simulink model "sampleModel1419"  (R2023a)
settings: Solver=VariableStepAuto  StartTime=0.0  StopTime=10.0  RelTol=1e-3
libraries: hdlsllib x6, simulink x1
settings Model: Creator=user1  LastModifiedBy=user1

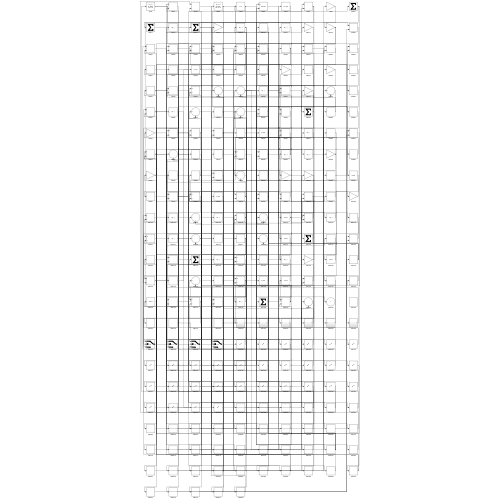
[thumbnail: Simulink's stored preview of the top-level diagram]
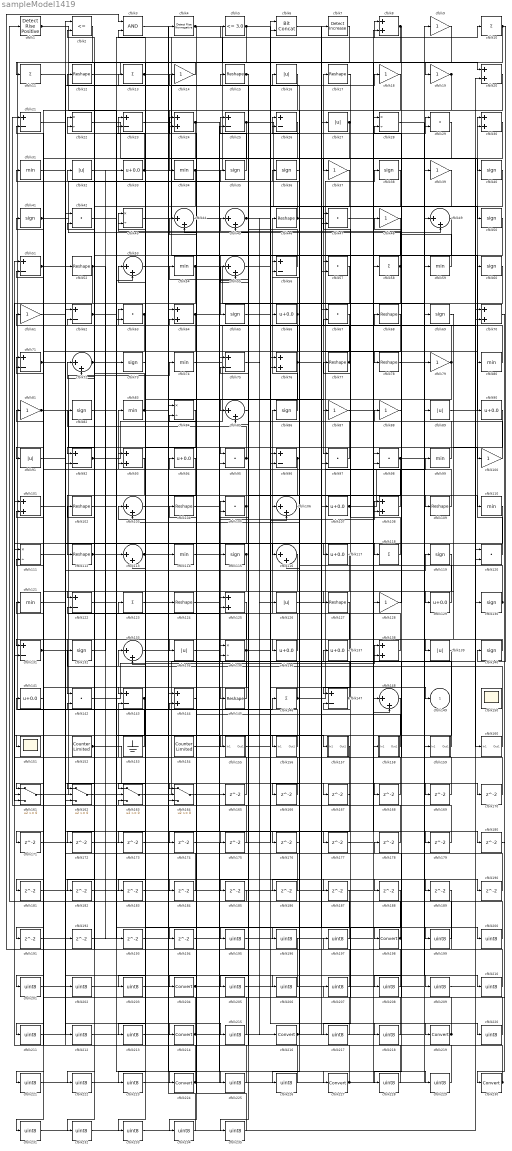
== system sampleModel1419 ==
  cfblk1 : hdlsllib/Logic and Bit Operations/Detect Rise Positive  vinit=0  OutDataTypeStr=boolean
  cfblk{10..11,13,58,118,123,146} (7 alike) : Sum  Inputs=+
  cfblk{9,14,18..19,37,39,48,61,79,81,87..88,100,128} (14 alike) : Gain
  cfblk{8,20,24,30,64,70,76,93,101,108,125,138,144} (13 alike) : Sum
  cfblk{12,15,17,46,52,68,77..78,102,104,109,112,124,127,145} (15 alike) : Reshape
  cfblk{44..45,49,53,55,72,85,103,106,113,116,133,148} (13 alike) : Sum  Inputs=|++
  cfblk{29,42,47,57,63,67,95,97..98,105,120,142} (12 alike) : DotProduct  OutDataTypeStr=Inherit: Inherit via internal rule
  cfblk{33,66,90,94,107,117,129,136..137,141} (10 alike) : Bias  Bias=0.0  SaturateOnIntegerOverflow=off
  cfblk{31,34,54,59,74,80,83,99,110,114,121} (11 alike) : MinMax
  cfblk{22,28,43,84,111,135} (6 alike) : Product  Inputs=*/  RndMeth=Zero  SaturateOnIntegerOverflow=on
  cfblk{35..36,38,40..41,50,60,65,69,73,82,86,115,119,130,132,140} (17 alike) : Signum
  cfblk{21,23,25..26,51,56,62,71,75,92,96,122,131,143,147} (15 alike) : Sum  Inputs=+-
  cfblk{16,27,32,89,91,126,134,139} (8 alike) : Abs  SaturateOnIntegerOverflow=off
  cfblk150 : Scope
      settings: Floating=on
  cfblk151 : Scope
  cfblk152 : hdlsllib/Sources/Counter Limited  uplimit=7  tsamp=-1
  cfblk153 : Ground
  cfblk154 : hdlsllib/Sources/Counter Limited  uplimit=7  tsamp=-1
  cfblk155 : Subsystem
      settings: LibrarySourceBlock=|
      | hdlsllib/Ports &
      | Subsystems/Subsystem
  cfblk156 : Subsystem
      settings: LibrarySourceBlock=|
      | hdlsllib/Ports &
      | Subsystems/Subsystem
  cfblk157 : Subsystem
      settings: LibrarySourceBlock=|
      | hdlsllib/Ports &
      | Subsystems/Subsystem
  cfblk158 : Subsystem
      settings: LibrarySourceBlock=|
      | hdlsllib/Ports &
      | Subsystems/Subsystem
  cfblk159 : Subsystem
      settings: LibrarySourceBlock=|
      | hdlsllib/Ports &
      | Subsystems/Subsystem
  cfblk160 : Subsystem
      settings: LibrarySourceBlock=|
      | hdlsllib/Ports &
      | Subsystems/Subsystem
  cfblk{161..164} (4 alike) : Switch  SaturateOnIntegerOverflow=off  InputSameDT=off
  cfblk{165..194} (30 alike) : Delay  SampleTime=1
  cfblk{195..197,199..203,205..213,215,217..218,220..223,225..226,228..229,231..235} (33 alike) : DataTypeConversion  OutDataTypeStr=uint8  SaturateOnIntegerOverflow=off  RndMeth=Floor
  cfblk{198,204,214,216,219,224,227,230} (8 alike) : DataTypeConversion  SaturateOnIntegerOverflow=off  RndMeth=Floor
  cfblk2 : RelationalOperator  Operator=<=  OutDataTypeStr=boolean  InputSameDT=off
  cfblk3 : Logic  AllPortsSameDT=off  OutDataTypeStr=boolean
  cfblk4 : hdlsllib/Logic and Bit Operations/Detect Rise Nonnegative  vinit=0  OutDataTypeStr=boolean
  cfblk5 : hdlsllib/Logic and Bit Operations/Compare To Constant  relop=<=  const=3.0  OutDataTypeStr=boolean
  cfblk6 : hdlsllib/Logic and Bit Operations/Bit Concat  numInputs=2
  cfblk7 : simulink/Logic and Bit Operations/Detect Increase  vinit=0.0  OutDataTypeStr=boolean
      settings: LibrarySourceBlock=|
      | hdlsllib/Logic and Bit
      | Operations/Detect
      | Increase
  cfblk149 : Outport  VectorParamsAs1DForOutWhenUnconnected=off
  wires:
  cfblk142/1 -> cfblk138/1
  cfblk30/1 -> cfblk156/1(In1)
  cfblk132/1 -> cfblk33/1
  cfblk146/1 -> cfblk38/1, cfblk94/1
  cfblk49/1 -> cfblk65/1
  cfblk43/1 -> cfblk10/1
  cfblk33/1 -> cfblk22/1, cfblk109/1
  cfblk15/1 -> cfblk45/2, cfblk205/1
  cfblk80/1 -> cfblk46/1
  cfblk46/1 -> cfblk18/1, cfblk21/2, cfblk199/1
  cfblk47/1 -> cfblk158/1(In1)
  cfblk50/1 -> cfblk97/1
  cfblk99/1 -> cfblk54/1
  cfblk89/1 -> cfblk30/1
  cfblk2/1 -> cfblk146/1
  cfblk37/1 -> cfblk57/1
  cfblk86/1 -> cfblk66/1
  cfblk113/1 -> cfblk35/1, cfblk167/1
  cfblk42/1 -> cfblk198/1
  cfblk145/1 -> cfblk103/1
  cfblk12/1 -> cfblk20/1
  cfblk120/1 -> cfblk30/2
  cfblk22/1 -> cfblk40/1
  cfblk34/1 -> cfblk8/1, cfblk92/1
  cfblk138/1 -> cfblk86/1
  cfblk147/1 -> cfblk105/1, cfblk122/2
  cfblk107/1 -> cfblk99/1, cfblk147/1
  cfblk105/1 -> cfblk83/1, cfblk131/2
  cfblk13/1 -> cfblk90/1, cfblk37/1
  cfblk109/1 -> cfblk47/1
  cfblk143/1 -> cfblk23/1, cfblk161/3
  cfblk18/1 -> cfblk34/1
  cfblk69/1 -> cfblk139/1
  cfblk158/1(Out1) -> cfblk64/2
  cfblk137/1 -> cfblk63/1
  cfblk126/1 -> cfblk49/1
  cfblk77/1 -> cfblk16/1, cfblk26/1
  cfblk7/1 -> cfblk204/1
  cfblk98/1 -> cfblk9/1, cfblk145/1
  cfblk8/1 -> cfblk228/1, cfblk232/1
  cfblk161/1 -> cfblk74/1
  cfblk83/1 -> cfblk61/1, cfblk87/1
  cfblk74/1 -> cfblk68/1
  cfblk35/1 -> cfblk25/1
  cfblk48/1 -> cfblk122/1
  cfblk38/1 -> cfblk63/2
  cfblk56/1 -> cfblk14/1
  cfblk140/1 -> cfblk134/1
  cfblk102/1 -> cfblk73/1
  cfblk14/1 -> cfblk11/1
  cfblk154/1 -> cfblk120/2
  cfblk134/1 -> cfblk108/1
  cfblk36/1 -> cfblk116/1
  cfblk63/1 -> cfblk13/1, cfblk191/1
  cfblk106/1 -> cfblk136/1
  cfblk10/1 -> cfblk140/1, cfblk19/1
  cfblk163/1 -> cfblk128/1
  cfblk41/1 -> cfblk49/2, cfblk4/1
  cfblk141/1 -> cfblk81/1
  cfblk71/1 -> cfblk169/1, cfblk170/1
  cfblk92/1 -> cfblk20/2, cfblk95/1, cfblk200/1
  cfblk58/1 -> cfblk45/1, cfblk95/2
  cfblk25/1 -> cfblk79/1, cfblk131/1
  cfblk131/1 -> cfblk115/1, cfblk119/1
  cfblk100/1 -> cfblk43/1
  cfblk127/1 -> cfblk142/1
  cfblk11/1 -> cfblk52/1
  cfblk95/1 -> cfblk155/1(In1), cfblk82/1
  cfblk4/1 -> cfblk106/2, cfblk194/1
  cfblk81/1 -> cfblk41/1, cfblk107/1
  cfblk62/1 -> cfblk157/1(In1), cfblk97/2
  cfblk79/1 -> cfblk143/1, cfblk24/2
  cfblk66/1 -> cfblk96/2, cfblk56/2
  cfblk117/1 -> cfblk162/1
  cfblk23/1 -> cfblk160/1(In1)
  cfblk108/1 -> cfblk71/1
  cfblk115/1 -> cfblk161/1, cfblk181/1
  cfblk70/1 -> cfblk230/1
  cfblk96/1 -> cfblk26/2, cfblk235/1
  cfblk57/1 -> cfblk85/1
  cfblk28/1 -> cfblk159/1(In1)
  cfblk144/1 -> cfblk224/1
  cfblk54/1 -> cfblk89/1, cfblk151/1
  cfblk31/1 -> cfblk214/1
  cfblk55/1 -> cfblk219/1
  cfblk40/1 -> cfblk47/2
  cfblk17/1 -> cfblk127/1
  cfblk112/1 -> cfblk113/1, cfblk164/3
  cfblk122/1 -> cfblk24/1
  cfblk19/1 -> cfblk85/2, cfblk186/1
  cfblk27/1 -> cfblk163/1, cfblk166/1
  cfblk159/1(Out1) -> cfblk15/1
  cfblk53/1 -> cfblk110/1
  cfblk124/1 -> cfblk67/2
  cfblk64/1 -> cfblk108/2, cfblk92/2, cfblk168/1
  cfblk45/1 -> cfblk149/1, cfblk126/1, cfblk50/1, cfblk220/1
  cfblk24/1 -> cfblk100/1, cfblk231/1
  cfblk152/1 -> cfblk164/1, cfblk2/2
  cfblk153/1 -> cfblk71/2
  cfblk118/1 -> cfblk77/1
  cfblk52/1 -> cfblk91/1, cfblk161/2, cfblk193/1
  cfblk75/1 -> cfblk216/1
  cfblk72/1 -> cfblk118/1, cfblk5/1
  cfblk93/1 -> cfblk112/1
  cfblk130/1 -> cfblk56/1, cfblk12/1, cfblk103/2
  cfblk73/1 -> cfblk113/2
  cfblk90/1 -> cfblk129/1
  cfblk76/1 -> cfblk164/2, cfblk62/2, cfblk78/1
  cfblk136/1 -> cfblk104/1
  cfblk9/1 -> cfblk76/2
  cfblk133/1 -> cfblk227/1
  cfblk6/1 -> cfblk80/1
  cfblk97/1 -> cfblk32/1
  cfblk110/1 -> cfblk135/2
  cfblk114/1 -> cfblk29/1
  cfblk160/1(Out1) -> cfblk132/1
  cfblk5/1 -> cfblk173/1, cfblk218/1
  cfblk51/1 -> cfblk117/1, cfblk17/1
  cfblk156/1(Out1) -> cfblk93/1
  cfblk157/1(Out1) -> cfblk21/1
  cfblk1/1 -> cfblk53/2, cfblk58/1
  cfblk59/1 -> cfblk28/2
  cfblk44/1 -> cfblk60/1
  cfblk128/1 -> cfblk88/1
  cfblk20/1 -> cfblk72/2
  cfblk135/1 -> cfblk6/2, cfblk162/3, cfblk102/1, cfblk221/1
  cfblk129/1 -> cfblk48/1
  cfblk164/1 -> cfblk165/1
  cfblk165/1 -> cfblk135/1
  cfblk166/1 -> cfblk51/1
  cfblk168/1 -> cfblk76/1
  cfblk169/1 -> cfblk138/2
  cfblk170/1 -> cfblk143/2
  cfblk16/1 -> cfblk171/1
  cfblk171/1 -> cfblk96/1
  cfblk26/1 -> cfblk172/1
  cfblk172/1 -> cfblk23/2
  cfblk173/1 -> cfblk6/1
  cfblk116/1 -> cfblk174/1
  cfblk60/1 -> cfblk175/1
  cfblk175/1 -> cfblk53/1
  cfblk29/1 -> cfblk176/1
  cfblk104/1 -> cfblk177/1
  cfblk177/1 -> cfblk98/2
  cfblk178/1 -> cfblk93/2
  cfblk61/1 -> cfblk179/1
  cfblk179/1 -> cfblk72/1
  cfblk87/1 -> cfblk180/1
  cfblk181/1 -> cfblk25/2
  cfblk68/1 -> cfblk182/1
  cfblk182/1 -> cfblk22/2
  cfblk119/1 -> cfblk183/1
  cfblk183/1 -> cfblk28/1
  cfblk111/1 -> cfblk184/1
  cfblk184/1 -> cfblk162/2
  cfblk85/1 -> cfblk185/1
  cfblk185/1 -> cfblk1/1
  cfblk186/1 -> cfblk43/2
  cfblk65/1 -> cfblk187/1
  cfblk32/1 -> cfblk188/1
  cfblk155/1(Out1) -> cfblk189/1
  cfblk82/1 -> cfblk190/1
  cfblk190/1 -> cfblk62/1
  cfblk191/1 -> cfblk163/2
  cfblk121/1 -> cfblk192/1
  cfblk192/1 -> cfblk64/1
  cfblk193/1 -> cfblk163/3
  cfblk194/1 -> cfblk8/2
  cfblk3/1 -> cfblk195/1
  cfblk195/1 -> cfblk27/1
  cfblk67/1 -> cfblk196/1
  cfblk196/1 -> cfblk3/1
  cfblk189/1 -> cfblk197/1
  cfblk197/1 -> cfblk3/2
  cfblk198/1 -> cfblk121/1, cfblk137/1
  cfblk199/1 -> cfblk42/1
  cfblk200/1 -> cfblk42/2
  cfblk125/1 -> cfblk201/1
  cfblk201/1 -> cfblk114/1
  cfblk91/1 -> cfblk202/1
  cfblk202/1 -> cfblk125/1
  cfblk94/1 -> cfblk203/1
  cfblk203/1 -> cfblk125/2
  cfblk204/1 -> cfblk29/2, cfblk44/1
  cfblk205/1 -> cfblk7/1
  cfblk101/1 -> cfblk206/1
  cfblk206/1 -> cfblk142/2
  cfblk180/1 -> cfblk207/1
  cfblk207/1 -> cfblk101/1
  cfblk88/1 -> cfblk208/1
  cfblk208/1 -> cfblk101/2
  cfblk123/1 -> cfblk209/1
  cfblk209/1 -> cfblk130/1
  cfblk78/1 -> cfblk210/1
  cfblk210/1 -> cfblk123/1
  cfblk148/1 -> cfblk211/1
  cfblk211/1 -> cfblk124/1
  cfblk21/1 -> cfblk212/1
  cfblk212/1 -> cfblk148/1
  cfblk187/1 -> cfblk213/1
  cfblk213/1 -> cfblk148/2
  cfblk214/1 -> cfblk141/1, cfblk67/1
  cfblk103/1 -> cfblk215/1
  cfblk215/1 -> cfblk31/1
  cfblk216/1 -> cfblk57/2, cfblk59/1, cfblk36/1
  cfblk188/1 -> cfblk217/1
  cfblk217/1 -> cfblk75/1
  cfblk218/1 -> cfblk75/2
  cfblk219/1 -> cfblk178/1, cfblk147/2, cfblk106/1, cfblk116/2
  cfblk220/1 -> cfblk55/1
  cfblk221/1 -> cfblk55/2
  cfblk39/1 -> cfblk222/1
  cfblk222/1 -> cfblk98/1
  cfblk139/1 -> cfblk223/1
  cfblk223/1 -> cfblk39/1
  cfblk224/1 -> cfblk111/1, cfblk44/2, cfblk69/1
  cfblk162/1 -> cfblk225/1
  cfblk225/1 -> cfblk144/1
  cfblk176/1 -> cfblk226/1
  cfblk226/1 -> cfblk144/2
  cfblk227/1 -> cfblk2/1, cfblk51/2
  cfblk228/1 -> cfblk133/1
  cfblk174/1 -> cfblk229/1
  cfblk229/1 -> cfblk133/2
  cfblk230/1 -> cfblk111/2, cfblk105/2
  cfblk231/1 -> cfblk70/1
  cfblk232/1 -> cfblk70/2
  cfblk84/1 -> cfblk233/1
  cfblk233/1 -> cfblk120/1
  cfblk167/1 -> cfblk234/1
  cfblk234/1 -> cfblk84/1
  cfblk235/1 -> cfblk84/2

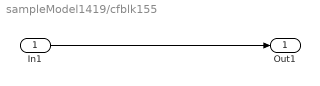
== system sampleModel1419/cfblk155 ==
  In1 : Inport
  Out1 : Outport
  wires:
  In1/1 -> Out1/1

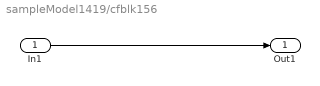
== system sampleModel1419/cfblk156 ==
  In1 : Inport
  Out1 : Outport
  wires:
  In1/1 -> Out1/1

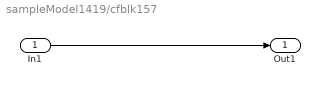
== system sampleModel1419/cfblk157 ==
  In1 : Inport
  Out1 : Outport
  wires:
  In1/1 -> Out1/1

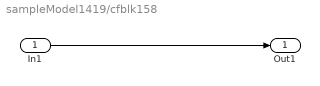
== system sampleModel1419/cfblk158 ==
  In1 : Inport
  Out1 : Outport
  wires:
  In1/1 -> Out1/1

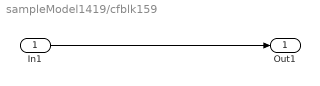
== system sampleModel1419/cfblk159 ==
  In1 : Inport
  Out1 : Outport
  wires:
  In1/1 -> Out1/1

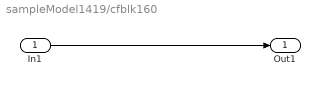
== system sampleModel1419/cfblk160 ==
  In1 : Inport
  Out1 : Outport
  wires:
  In1/1 -> Out1/1
